simulink model "validacion_subsistema_termico"  (R2023b)
settings: Solver=VariableStepAuto  StartTime=0.0  StopTime=10.0  RelTol=1e-3
values from neighbouring files (symbols this model uses):
  alpha_Cu = 3.9e-3    (= 0.0039)    [controlador_foc_simulink.m]    (also in parametros_planta.m; params_subsistema_termico.m; sistema_completo_en_codigo.m)
  Cts = 0.818    [parametros_planta.m]    (also in params_subsistema_termico.m)
  ia_test = 0.565    [plot_validacion_subsistema_termico.m]
  ib_test = -0.2825    [plot_validacion_subsistema_termico.m]
  ic_test = -0.2825    [plot_validacion_subsistema_termico.m]
  Rs_REF = 1.02    [controlador_foc_simulink.m]    (also in parametros_planta.m; params_subsistema_termico.m; sistema_completo_en_codigo.m)
  Rts_amb = 146.7    [parametros_planta.m]    (also in params_subsistema_termico.m)
  Ts_REF = 20.0    (= 20)    [controlador_foc_simulink.m]    (also in parametros_planta.m; params_subsistema_termico.m; sistema_completo_en_codigo.m)
undefined symbols (not defined in the file or in its folder): Tamb_test
settings Model: Creator=Pc  LastModifiedBy=Pc

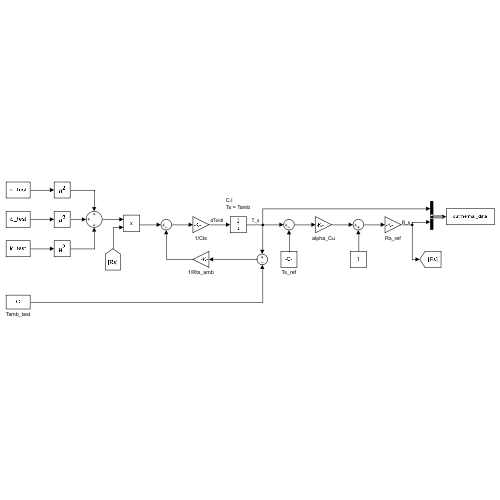
[thumbnail: Simulink's stored preview of the top-level diagram]
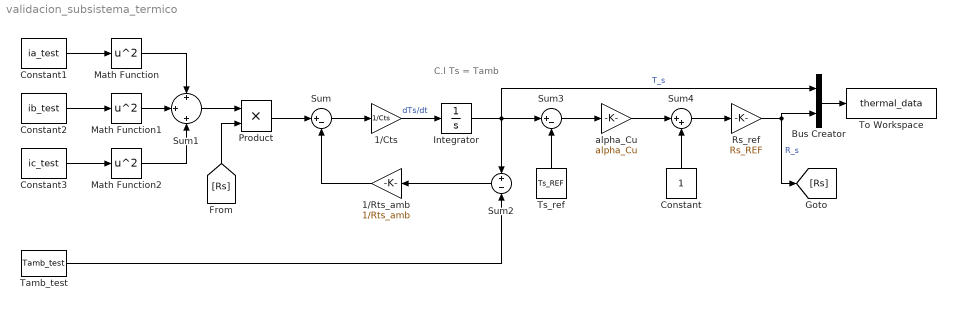
== system validacion_subsistema_termico ==
  note: C.l
      | Ts = Tamb
  1/Cts : Gain  Gain=1/Cts
  1/Rts_amb : Gain  Gain=1/Rts_amb
  Bus Creator : BusCreator  Inputs=2
  Constant : Constant
  Constant1 : Constant  Value=ia_test
  Constant2 : Constant  Value=ib_test
  Constant3 : Constant  Value=ic_test
  Integrator : Integrator  InitialCondition=Tamb_test
  Math Function : Math  Operator=square
  Math Function1 : Math  Operator=square
  Math Function2 : Math  Operator=square
  Product : Product
  Rs_ref : Gain  Gain=Rs_REF
  Sum : Sum  Inputs=|+-
  Sum1 : Sum  Inputs=+|+|+
  Sum2 : Sum  Inputs=+-
  Sum3 : Sum  Inputs=|+-
  Sum4 : Sum  Inputs=|++
  Tamb_test : Constant  Value=Tamb_test
  To Workspace : ToWorkspace  VariableName=thermal_data  SaveFormat=Timeseries  SampleTime=-1
  Ts_ref : Constant  Value=Ts_REF
  alpha_Cu : Gain  Gain=alpha_Cu
  wires:
  1/Cts/1 -> Integrator/1  "dTs/dt"
  Sum/1 -> 1/Cts/1
  Integrator/1 -> Bus Creator/1, Sum2/1, Sum3/1  "T_s"
  Math Function/1 -> Sum1/1
  Math Function1/1 -> Sum1/2
  Math Function2/1 -> Sum1/3
  Sum1/1 -> Product/1
  Product/1 -> Sum/1
  1/Rts_amb/1 -> Sum/2
  Sum2/1 -> 1/Rts_amb/1
  Ts_ref/1 -> Sum3/2
  Sum3/1 -> alpha_Cu/1
  alpha_Cu/1 -> Sum4/1
  Constant/1 -> Sum4/2
  Sum4/1 -> Rs_ref/1
  Rs_ref/1 -> Bus Creator/2, [Rs]  "R_s"
  [Rs] -> Product/2
  Constant1/1 -> Math Function/1
  Constant3/1 -> Math Function2/1
  Constant2/1 -> Math Function1/1
  Tamb_test/1 -> Sum2/2
  Bus Creator/1 -> To Workspace/1
